simulink model "ContoleLateralApplication_atual"  (R2021a)
settings: Solver=ode23tb  StartTime=0.0  StopTime=TME.Simulation  FixedStep=.001  RelTol=1e-3  EnableMultiTasking=on
StartFcn:
  | %tic
StopFcn:
  | %toc
model workspace (MAT data in the model file):
  A_mu = 10
  B_reff = 8.386
  Cz = 7766.25
  DCT_Param.Transmission.Ratios = [3.78 2.18 1.43 1.03 0.935 0.84]
  DCT_Param.Transmission.Shaft_Inertia_Odd = 0.0023
  DCT_Param.Transmission.Shaft_Inertia_Even = 0.0009
  DCT_Param.Transmission.Shaft_Inertia_Output = 0.008
  DCT_Param.Transmission.Gear_Inertia = 0.001
  DCT_Param.Transmission.Gear_Efficiency = 0.94
  DCT_Param.Transmission.Gear_Ang_Vel_Thr = 0.01
  DCT_Param.Transmission.Shaft_Velocity_Odd = 0
  DCT_Param.Transmission.Shaft_Velocity_Even = 0
  DCT_Param.Transmission.Shaft_Velocity_Output = 0
  DCT_Param.Transmission.Gear_Initial_Velocity = 0
  DCT_Param.Transmission.Abstract.Compliance = 100000
  DCT_Param.Transmission.Abstract.Damping = 10000
  DCT_Param.Transmission.Abstract.Ratio_Time_Const = 0.05
  DCT_Param.Transmission.Abstract.Shift_Gear_Delay = 25
  DCT_Param.Clutch.Torque_Radius = 130
  DCT_Param.Clutch.Num_Friction_Surfaces = 4
  DCT_Param.Clutch.Engagement_Piston_Area = 0.001
  DCT_Param.Clutch.Kinetic_Friction_Coeff = 0.3
  DCT_Param.Clutch.Static_Friction_Coeff = 0.31
  DCT_Param.Clutch.Derating_Factor = 1
  DCT_Param.Clutch.Clutch_Velocity_Tolerance = 0.001
  DCT_Param.Clutch.Threshold_Pressure = 1
  DCT_Param.Clutch.Drag_Torque_Coeff = 0
  DCT_Param.Dog_Clutch.Max_Torque = 1000
  DCT_Param.Dog_Clutch.Teeth_Mean_Radius = 50
  DCT_Param.Dog_Clutch.Tooth_Height = 10
  DCT_Param.Dog_Clutch.Ring_Hub_Clearance = 3
  DCT_Param.Dog_Clutch.Ring_Stop_Stiffness = 1000000
  DCT_Param.Dog_Clutch.Ring_Stop_Damping = 1000
  DCT_Param.Dog_Clutch.Shift_Linkage_Damping = 100
  DCT_Param.Dog_Clutch.Max_Engage_Velocity = 1000000
  DCT_Param.Dog_Clutch.Tooth_Engage_Overlap = 3
  DCT_Param.Vehicle.Mass = 1600
  DCT_Param.Vehicle.Wheels_Per_Axle = 2
  DCT_Param.Vehicle.Distance_CG_FrontAxle = 1.7
  DCT_Param.Vehicle.Distance_CG_RearAxle = 2
  DCT_Param.Vehicle.Distance_CG_Ground = 0.5
  DCT_Param.Vehicle.Frontal_Area = 3
  DCT_Param.Vehicle.Aero_Drag_Coeff = 0.4
  DCT_Param.Vehicle.Initial_Velocity = 0
  DCT_Param.Vehicle.Final_Drive_Ratio = 3.7
  DCT_Param.Vehicle.Final_Drive_Efficiency = 0.86
  DCT_Param.Vehicle.Final_Drive_Vel_Thresh = 0.01
  DCT_Param.Vehicle.Side_Shaft_Inertia = 0.01
  DCT_Param.Vehicle.Side_Shaft_Initial_Velocity = 0
  DCT_Param.Vehicle.Tire.Radius = 0.312
  DCT_Param.Vehicle.Tire.Inertia = 0.5
  DCT_Param.Vehicle.Tire.Initial_Velocity = 0
  DCT_Param.Vehicle.Tire.Slip_Vel_Thresh = 0.1
  DCT_Param.Vehicle.Tire.Nominal_Vertical_Load = 4000
  DCT_Param.Vehicle.Tire.C_Coeff = 1.685
  DCT_Param.Vehicle.Tire.D_Coeff = [1.21 -0.037]
  DCT_Param.Vehicle.Tire.E_Coeff = [0.344 0.095 -0.02 0]
  DCT_Param.Vehicle.Tire.BCD_Coeff = [21.51 -0.163 0.245]
  DCT_Param.Vehicle.Tire.H_Coeff = [-0.002 0.002]
  DCT_Param.Vehicle.Tire.V_Coeff = [0 0]
  DCT_Param.ICE.Max_Power = 100000
  DCT_Param.ICE.Speed_At_Max_Power = 5500
  DCT_Param.ICE.Max_Speed = 7000
  DCT_Param.ICE.Stall_Speed = 200
  DCT_Param.ICE.Shaft_Inertia = 0.2
  DCT_Param.ICE.Initial_Velocity = 800
  DCT_Param.ICE.Idle_Ref_Spd = 800
  DCT_Param.ICE.Engine_Time_Constant = 0.2
  DCT_Param.ICE.Initial_Normalized_Throttle = 0
  DCT_Param.ICE.Speed_Threshold = 20
  DCT_Param.ICE.FC.Speed_Vector = [0 368.421052632 736.842105263 1105.26315789 1473.68421053 1842.10526316 2210.52631579 2578.94736842 2947.36842105 3315.78947368 3684.21052632 4052.63157895 4421.05263158 4789.47368421 5157.89473684 5526.31578947 5894.73684211 6263.15789474 6631.57894737 7000]
  DCT_Param.ICE.FC.Torque_Vector = [0 10.5263157895 21.0526315789 31.5789473684 42.1052631579 52.6315789474 63.1578947368 73.6842105263 84.2105263158 94.7368421053 105.263157895 115.789473684 126.315789474 136.842105263 147.368421053 157.894736842 168.421052632 178.947368421 189.473684211 200]
  DCT_Param.ICE.FC.Consumption_Table = [0.262945178015 0.225304787522 0.201465019624 0.191425874321 0.195187351614 0.212749451502 0.244112173984 0.289275519063 0.348239486736 0.421004077004 0.507569289868 0.607935125326 ... (400 elements, 20x20)]
  DCT_Param.Shift_Map_Example.Pedal_Positions = [0.1 0.4 0.5 0.9]
  DCT_Param.Shift_Map_Example.Upshift_Speeds = [11  20  26  34.5  43; 14  26  35  44.5  55; 17  31  42  52.5  65; 21  39  52  66.5  80]
  DCT_Param.Shift_Map_Example.Downshift_Speeds = [8.9  17  23.6  32.4  40.8; 11.5  22.7  32  41.6  52.2; 14  27  38.1  50  62; 18  33  48  62.6  76.2]
  DCT_Param.Shift_Map_ORIG.Pedal_Positions = [0.1 0.4 0.5 0.9]
  DCT_Param.Shift_Map_ORIG.Upshift_Speeds = [11.5  23.5  35.5  45.5  55.5; 14.5  26.5  38.5  48.5  58.5; 17.5  29.5  41.5  51.5  61.5; 20.5  32.5  44.5  54.5  64.5]
  DCT_Param.Shift_Map_ORIG.Downshift_Speeds = [8.5  20.5  32.5  42.5  52.5; 11.5  23.5  35.5  45.5  55.5; 14.5  26.5  38.5  48.5  58.5; 17.5  29.5  41.5  51.5  61.5]
  DCT_Param.Shift_Map_OPT.Pedal_Positions = [0.1 0.4 0.5 0.9]
  DCT_Param.Shift_Map_OPT.Upshift_Speeds = [17.8469  29.8469  35.8159  41.2981  46.3004; 19.2469  33.9778  43.9778  53.9778  63.9778; 24.5469  41.9778  62.1778  78.5778  106.9778; 27.5469  59.3778  99.0445  109.0445  119.0445]
  DCT_Param.Shift_Map_OPT.Downshift_Speeds = [14.8469  26.8469  32.8159  38.2981  43.3004; 16.2469  30.9778  40.9778  50.9778  60.9778; 21.5469  38.9778  59.1778  75.5778  103.9778; 24.5469  56.3778  96.0445  106.0445  116.0445]
  DCT_Param.Shift_Map.Pedal_Positions = [0.1 0.4 0.5 0.9]
  DCT_Param.Shift_Map.Upshift_Speeds = [11.5  23.5  35.5  45.5  55.5; 14.5  26.5  38.5  48.5  58.5; 17.5  29.5  41.5  51.5  61.5; 20.5  32.5  44.5  54.5  64.5]
  DCT_Param.Shift_Map.Downshift_Speeds = [8.5  20.5  32.5  42.5  52.5; 11.5  23.5  35.5  45.5  55.5; 14.5  26.5  38.5  48.5  58.5; 17.5  29.5  41.5  51.5  61.5]
  DCT_Param.Control.Clutch.Min_Lock_Pressure = 2000000
  DCT_Param.Control.Clutch.Max_Lock_Pressure = 5000000
  DCT_Param.Control.Clutch.Max_Unlock_Pressure = 500000
  DCT_Param.Control.Engine_Start_RPM = 800
  DCT_Param.Control.Engine_Stop_RPM = 790
  DCT_Param.Control.Mode_Logic_TS = 0.1
  DCT_Param.Control.ICE.Kp = 0.02
  DCT_Param.Control.ICE.Ki = 0.01
  DCT_Param.Control.Gen.Kp = 10
  DCT_Param.Control.Gen.Ki = 3
  DCT_Param.Control.Mot.Kp = 500
  DCT_Param.Control.Mot.Ki = 300
  DCT_Param.Control.Veh_Spd.Kp = 0.02
  DCT_Param.Control.Veh_Spd.Ki = 0.04
  DCT_Param.Driver.Kp = 400
  DCT_Param.Driver.Ki = 0.001
  DCT_Param.Driver.Pedal_Filter_Const = 0.01
  DCT_Param.Dog_Clutches.Pulse_Delay = 50
  DCT_Param.Dog_Clutches.Pulse_Length = 20
  DCT_Param.Animation.Teeth_Ratios = [0.338461538462 0.555555555556 0.916666666667 0.96 1.17948717949 1.92307692308]
  DCT_Param.Animation.Teeth_Ratios_Reverse = [0.458333333333 0.75]
  DCT_Param.Shift_Map_OPT506.Pedal_Positions = [0.1 0.4 0.5 0.9]
  DCT_Param.Shift_Map_OPT506.Upshift_Speeds = [18  30.2  48.3  67.3322  77.3429; 20.1  36.85  66.6178  76.7537  86.7537; 21.1  40.25  71.0189  81.0189  91.7873; 24.1  63.75  80.7523  105.9489  115.9489]
  DCT_Param.Shift_Map_OPT506.Downshift_Speeds = [15  27.2  45.3  64.3322  74.3429; 17.1  33.85  63.6178  73.7537  83.7537; 18.1  37.25  68.0189  78.0189  88.7873; 21.1  60.75  77.7523  102.9489  112.9489]
  DCT_Param.Shift_Map_OPTAbsRea176.Pedal_Positions = [0.1 0.4 0.5 0.9]
  DCT_Param.Shift_Map_OPTAbsRea176.Upshift_Speeds = [17.8469  29.8469  35.7875  44.0901  49.4243; 18.9219  34.1312  45.8256  59.7585  69.7585; 32.1719  43.4585  53.51  103.2151  114.6401; 35.1719  59.2585  99.5217  109.5217  119.5217]
  DCT_Param.Shift_Map_OPTAbsRea176.Downshift_Speeds = [14.8469  26.8469  32.7875  41.0901  46.4243; 15.9219  31.1312  42.8256  56.7585  66.7585; 29.1719  40.4585  50.51  100.2151  111.6401; 32.1719  56.2585  96.5217  106.5217  116.5217]
  DLCXref = [0 6 7 14 33.5 34 42 50 60]
  DLCYref = [0 0 -4.5 -4 -3.75 1.5 0.5 0 0]
  D_reff = 0.25826
  Downshift_Speeds = [9.5625  23.0625  36.5625  47.8125  59.0625  68.90625  78.75; 12.9375  26.4375  39.9375  51.1875  62.4375  72.84375  83.25; 16.3125  29.8125  43.3125  54.5625  65.8125  76.78125  87.75; 19.6875  33.1875  46.6875  57.9375  69.1875  80.71875  92.25]
  EngRevLim = 7000
  Pedal_Positions = [0.1 0.4 0.5 0.9]
  SUS.Stiffness = 24000
  SUS.Damping.Constant = 1262
  SUS.Damping.Rebound = [4040 4950 2883 2043]
  SUS.Damping.Compression = [3600 3420 1863 1472]
  SUS.PistonSpeed = [0.05 0.1 0.3 0.6]
  SUS.UnsprungMass.Fr = 21.0693333333
  SUS.UnsprungMass.Rr = 21.0693333333
  Upshift_Speeds = [12.9375  26.4375  39.9375  51.1875  62.4375  72.84375  83.25; 16.3125  29.8125  43.3125  54.5625  65.8125  76.78125  87.75; 19.6875  33.1875  46.6875  57.9375  69.1875  80.71875  92.25; 33  52.5  77.25  100.5  138.75  161.875  185]
  VEH.Mass = 1181
  VEH.StaticNormalFrontLoad.FR = 264.666666667
  VEH.StaticNormalFrontLoad.FL = 264.666666667
  VEH.StaticNormalRearLoad.RR = 322
  VEH.StaticNormalRearLoad.RL = 322
  VEH.WheelBase = 3.075
  VEH.FrontAxlePositionfromCG = 1.515
  VEH.RearAxlePositionfromCG = 1.504
  VEH.HeightCG = 0.134
  VEH.FrontalArea = 2.11
  VEH.DragCoefficient = 0.33
  VEH.NumberOfWheelsPerAxle = 2
  VEH.Thread.FR = 1.705
  VEH.Thread.RR = 1.705
  VEH.PitchMomentInertia = 1922.66666667
  VEH.RollMomentInertia = 432.333333333
  VEH.YawMomentInertia = 2066
  VEH.SteeringRatio = 18
  VEH.TrackWidth = 1.922
  VEH.SprungMass = 1096.72266667
  VEH.InitialLongPosition = 0
  VEH.InitialLatPosition = 0
  VEH.InitialVertPosition = 0
  VEH.InitialRollAngle = 0
  VEH.InitialPitchAngle = 0
  VEH.InitialYawAngle = 0
  VEH.InitialLongVel = 0
  VEH.InitialLatVel = 0
  VEH.InitialVertVel = 0
  VEH.InitialRollRate = 0
  VEH.InitialPitchRate = 0
  VEH.InitialYawRate = 0
  V_o = 16.7
  V_xlow = 1
  WH.Tire.Radius.Front = 0.384
  WH.Tire.Radius.Rear = 0.401
  WH.Tire.Sidewall = 0.245
  WH.Tire.RollingResistCoeff = 0.0103
  WH.Tire.Magic.B = 10
  WH.Tire.Magic.C = 1.9
  WH.Tire.Magic.D = 1
  WH.Tire.Magic.E = 0.97
  WH.Tire.Magic.Bx = 12
  WH.Tire.Magic.Cx = 1.9
  WH.Tire.Magic.Dx = 0.72
  WH.Tire.Magic.Ex = 0.95
  WH.Tire.Magic.By = 12
  WH.Tire.Magic.Cy = 1.3
  WH.Tire.Magic.Dy = 0.75
  WH.Tire.Magic.Ey = 0.2
  WH.Tire.Front.Ky = 40000
  WH.Tire.Rear.Ky = 40000
  WH.Tire.Kz = 320000
  WH.Tire.Damping = 100
  WH.Inertia = 1.00333333333
  WH.Mass = 11.4333333333
  WH.DampingCoefficient = 0.01
  WH.VelocityTol = 0.1
  a = 1.4
  alpha_max = 1.5
  alpha_min = -1.5
  b = 1.8
  c_zo = 209651
  epsilon = 0.1
  h = 0.134
  path.ISO3888p2.x = [0 2 12 25.5 36.5 49 61]
  path.ISO3888p2.y = [0 0 0 3.725 3.725 0 0]
  path.ISO3888p2.ylb = [1.225 1.225 1.225 4.725 4.725 1.5 1.5]
  path.ISO3888p2.yrb = [-1.225 -1.225 -1.225 2.225 2.225 -1.5 -1.5]
  path.CUSC.x = [10.668 21.336 36.576 54.864 73.152]
  path.CUSC.y = [0 0 5.1816 0 0]
  path.CUSC.ylb = [1.2192 1.2192 7.0104 1.8288 1.8288]
  path.CUSC.yrb = [-1.2192 -1.2192 3.3528 -1.8288 -1.8288]
  pio = 220000
  q_Fcx = 0
  q_Fz2 = 15.4
  q_Fzy = 0
  q_reo = 0.9974
  q_sx1 = -0.007764
  q_sx10 = 0.2824
  q_sx11 = 5.349
  q_sx12 = 0
  q_sx13 = 0
  q_sx14 = 0
  q_sx2 = 1.1915
  q_sx3 = 0.013948
  q_sx4 = 4.912
  q_sx5 = 1.02
  q_sx6 = 22.83
  q_sx7 = 0.7104
  q_sx8 = -0.023393
  q_sx9 = 0.6581
  q_sy1 = 0.00702
  q_sy2 = 0
  q_sy3 = 0.001515
  q_sy4 = 8.514e-05
  q_sy5 = 0
  q_sy6 = 0
  q_sy7 = 0.9008
  q_sy8 = -0.4089
  q_v1 = 0.0007742
  q_v2 = 0.04667
  r_Bx1 = 12.531
  r_Bx2 = 9.532
  r_Bx3 = 0
  r_By1 = 10.615
  r_By2 = 7.705
  r_By3 = 3.433e-06
  r_By4 = 0
  r_Cx1 = 1.019
  r_Cy1 = 1.0585
  r_Ex1 = -0.4487
  r_Ex2 = -0.4726
  r_Ey1 = 0.3132
  r_Ey2 = 7.63e-06
  r_Hx1 = 0.0002374
  r_Hy1 = 0.011646
  r_Hy2 = 7.63e-06
  r_Vy1 = 0.05654
  r_Vy2 = 7.63e-06
  r_Vy3 = 0
  r_Vy4 = 99.9
  r_Vy5 = 2
  r_Vy6 = 15.814
  r_o = 0.3135
  vehWidth = 2
  w = 1
values from neighbouring files (symbols this model uses):
  C1 = 1.2801    [Data_ControleLateral_atual.m]
  C2 = 23.99    [Data_ControleLateral_atual.m]
  C3 = 0.52    [Data_ControleLateral_atual.m]
undefined symbols (not defined in the file or in its folder): Disabled, EV, GND, MTR, Right, SENSOR, STEER, WHL
libraries: autolibutils x5, vehdynlibscenariocommon x5, autolibshared x5, sim3dlib x4, vehdynlibtirecommon x2, autolibmappedmotor x2, vehdynlibviscommon x2, vehdynlibsteering x1, pid_lib x1, vehdynlibdriver x1, vehdynlibsens x1, sharedtransform x1
(part 1 of 6)
settings Model: SimulationMode=accelerator  NumberOfSteps=10  OrderedModelArguments=off  Creator=The MathWorks, Inc.  LastModifiedBy=Luiza
settings SolverCC: ZeroCrossAlgorithm=Adaptive  AlgebraicLoopSolver=TrustRegion  AutoInsertRateTranBlk=on  InsertRTBMode=Never (minimum delay)  DecoupledContinuousIntegration=on  MinimalZcImpactIntegration=on
settings OptimizationCC: EfficientMapNaN2IntZero=off
settings DebuggingCC: SignalInfNanChecking=error  ArtificialAlgebraicLoopMsg=none  MaskedZcDiagnostic=none  IgnoredZcDiagnostic=none  ModelReferenceExtraNoncontSigs=none  PregeneratedLibrarySubsystemCodeDiagnostic=none  SFMachineParentedDataDiag=warning  ArithmeticOperatorsInVariantConditions=warning
settings HardwareCC: TargetBitPerPointer=64  TargetBitPerSizeT=64  TargetBitPerPtrDiffT=64  TargetLongLongMode=on  TargetIntDivRoundTo=Zero  TargetEndianess=LittleEndian  TargetWordSize=64  TargetHWDeviceType=MATLAB Host  ProdEqTarget=off
settings ModelReferenceCC: UpdateModelReferenceTargets=IfOutOfDate  EnableParallelModelReferenceBuilds=on  ModelReferenceMinAlgLoopOccurrences=on  PropagateSignalLabelsOutOfModel=off
settings SFSimCC: SimUseLocalCustomCode=off  CustomCodeUndefinedFunction=UseInterfaceOnly
settings CodeAppCC: MaxIdLength=128
settings GRTTargetCC: TargetLangStandard=C89/C90 (ANSI)  CombineOutputUpdateFcns=off  GRTInterface=on

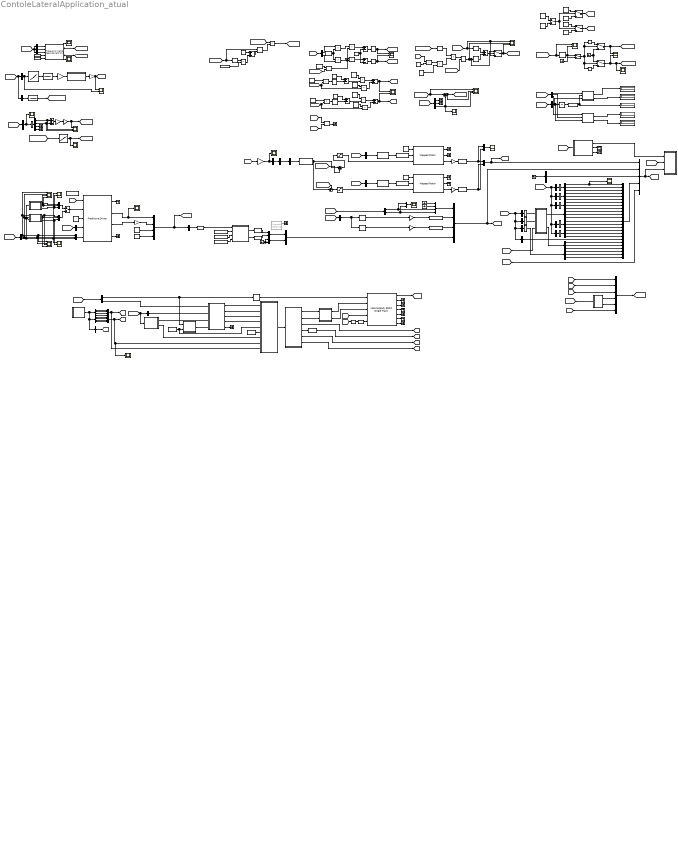
== system ContoleLateralApplication_atual ==
  note: Pista
  note: Avaliação
  note: Skid Pad / Slalom
  note: Steering System
  note: Driveline
  note: Powertrain
  note: Copyright 2018 The MathWorks, Inc.
  note: Copyright 2017-2018 The MathWorks, Inc.
  note: Taxa de guinada máxima
  note: Diferença entre guinadas
  note: GUINADA DESEJADA
      |
      | Variaveis necessárias:
      | Velocidade CG (vCG) - gps; velo. média rodas dianteiras (OK)
      | Lr + Lf - distancia entre os eixos traseiro e frontal (OK)
      | Ku - taxa de guinada desejada (OK)
      | Cy,f / Cy,r - rigidez dos pneus dianteiros e traseiros na curva (OK)
      | m - massa (OK)
      | Delta minusculo - angulo direçao (OK)
      |
      | GUINADA MÁXIMA
      |
      | Sigma: fator de ajustabilidade; necessita de teste para definido, varia cm o pavimento
      | Micro g: coeficiente de atrito (padrao);
      | vCG : velo, centro de gravidade
  note: Taxa de guinada desejada
  note: Variáveis
  note: ControladorVT
  note: APPS
  note: IMU
  note: Volante
  note: Sensores
  note: Coeficiente de atrito
  note: SLIP RATIO
      |
      | COEFICIENTE DE ATRITO
  Abs{,1..5} (6 alike) : Abs
  Acc to Torque Request : Gain  Gain=MTR.MaxTorque*0.01
  AccelCmd% : Gain  Gain=100
  Accelerometer : Scope
  Add : Sum
  Add1 : Sum
  Add{2..8} (7 alike) : Sum  Inputs=+-
  AngVolante-> AngRoda : Lookup_n-D  NumberOfTableDimensions=1  BreakpointsForDimension1=STEER.Volante  Table=SENSOR.SteerAvg  InternalRulePriority=Speed  RndMeth=Simplest  InputSameDT=on
  Axle Forces : Subsystem  Variant=on  VariantControlMode=label  LabelModeActiveChoice=1
  Bus Creator : BusCreator  Inputs=25
  Bus Creator1 : BusCreator  Inputs=4
  Bus Creator10 : BusCreator  Inputs=1
  Bus Creator11 : BusCreator  Inputs=4
  Bus Creator13 : BusCreator  Inputs=2
  Bus Creator2 : BusCreator  Inputs=5
  Bus Creator3 : BusCreator  Inputs=6
  Bus Creator4 : BusCreator  Inputs=1
  Bus Creator5 : BusCreator  Inputs=2
  Bus Creator9 : BusCreator  Inputs=1
  Bus Selector : BusSelector  OutputSignals=ECU.EngTrqCmd
  Bus Selector1 : BusSelector  OutputSignals=InertFrm.Cg.Disp.X,InertFrm.Cg.Disp.Y,InertFrm.Cg.Disp.Z  OutputAsBus=on
  Bus Selector10 : BusSelector  OutputSignals=Gnd.z.G_FL_z,Gnd.z.G_FR_z,Gnd.z.G_RL_z,Gnd.z.G_RR_z
  Bus Selector11 : BusSelector  OutputSignals=Wind
  Bus Selector12 : BusSelector  OutputSignals=Gnd.mu.mu_FL,Gnd.mu.mu_FR,Gnd.mu.mu_RL,Gnd.mu.mu_RR
  Bus Selector13 : BusSelector  OutputSignals=WhlAng,AxlTrq
  Bus Selector14 : BusSelector  OutputSignals=Steer
  Bus Selector15 : BusSelector  OutputSignals=omega
  Bus Selector16 : BusSelector  OutputSignals=BdyFrm.Cg.AngVel.r
  Bus Selector17 : BusSelector  OutputSignals=LeftMtrTrq,RghtMtrTrq
  Bus Selector18 : BusSelector  OutputSignals=LeftMtrSpd
  Bus Selector19 : BusSelector  OutputSignals=RghtMtrSpd
  Bus Selector2 : BusSelector  OutputSignals=InertFrm.Cg.Vel.Xdot,InertFrm.Cg.Vel.Ydot,InertFrm.Cg.Vel.Zdot  OutputAsBus=on
  Bus Selector20 : BusSelector  OutputSignals=Chassis.psi,Chassis.Y,Chassis.X
  Bus Selector21 : BusSelector  OutputSignals=LeftMtrSpd,RghtMtrSpd
  Bus Selector23 : BusSelector  OutputSignals=Steer
  Bus Selector25 : BusSelector  OutputSignals=Accel
  Bus Selector26 : BusSelector  OutputSignals=BdyFrm.Cg.Vel.xdot
  Bus Selector27 : BusSelector  OutputSignals=BdyFrm.Cg.AngVel  OutputAsBus=on
  Bus Selector28 : BusSelector  OutputSignals=BdyFrm.Cg.Acc.ax,BdyFrm.Cg.Acc.ay,BdyFrm.Cg.Acc.az  OutputAsBus=on
  Bus Selector29 : BusSelector  OutputSignals=BdyFrm.Cg.Acc.xddot,BdyFrm.Cg.Acc.yddot,BdyFrm.Cg.Acc.zddot  OutputAsBus=on
  Bus Selector3 : BusSelector  OutputSignals=BdyFrm.Cg.Acc.ax,BdyFrm.Cg.Acc.ay,BdyFrm.Cg.Acc.az  OutputAsBus=on
  Bus Selector31 : BusSelector  OutputSignals=Chassis.X,Chassis.Y,Chassis.psi
  Bus Selector32 : BusSelector  OutputSignals=omega
  Bus Selector33 : BusSelector  OutputSignals=BdyFrm.Cg.Vel.xdot  OutputAsBus=on
  Bus Selector4 : BusSelector  OutputSignals=InertFrm.Cg.Ang.phi,InertFrm.Cg.Ang.theta,InertFrm.Cg.Ang.psi  OutputAsBus=on
  Bus Selector5 : BusSelector  OutputSignals=BdyFrm.Cg.AngVel.p,BdyFrm.Cg.AngVel.q,BdyFrm.Cg.AngVel.r  OutputAsBus=on
  Bus Selector6 : BusSelector  OutputSignals=InertFrm.Geom.Disp.X,InertFrm.Geom.Disp.Y,InertFrm.Geom.Disp.Z  OutputAsBus=on
  Bus Selector7 : BusSelector  OutputSignals=InertFrm.Geom.Vel.Xdot,InertFrm.Geom.Vel.Ydot,InertFrm.Geom.Vel.Zdot  OutputAsBus=on
  Bus Selector8 : BusSelector  OutputSignals=BdyFrm.Geom.Ang.Beta
  Bus Selector9 : BusSelector  OutputSignals=BdyFrm.Cg.Vel.xdot,BdyFrm.Cg.Vel.ydot,BdyFrm.Cg.Vel.zdot  OutputAsBus=on
  Bus to Vector{,1..8} (9 alike) : BusToVector
  Constant : Constant  Value=76
  Constant1 : vehdynlibtirecommon/Constant  const=180000  numWheels=4
      settings: SourceProductBaseCode=VE
  Constant10 : Constant  Value=C3
  Constant11 : Constant  Value=STEER.Volante
  Constant12 : Constant  Value=STEER.Left
  Constant13 : Constant  Value=[0 0 0]
  Constant14 : Constant  Value=0
  Constant15 : Constant  Value=100
  Constant16 : Constant  Value=[0 0 9.78]
  Constant17 : Constant
  Constant18 : Constant  Value=C3
  Constant19 : Constant
  Constant2 : Constant  Value=76
  Constant20 : Constant  Value=C1
  Constant21 : Constant  Value=EV.InitialLongVel
  Constant22 : Constant  Value=0
  Constant23 : Constant  Value=-C2
  Constant24 : Constant  Value=9.1
  Constant25 : Constant  Value=1.3
  Constant26 : Constant  Value=1.1
  Constant27 : Constant  Value=8.7
  Constant3 : vehdynlibtirecommon/Constant  const=0  numWheels=4
      settings: SourceProductBaseCode=VE
  Constant4 : Constant  Value=2*pi/60
  Constant5 : Constant  Value=0.2566
  Constant6 : Constant
  Constant7 : Constant  Value=C1
  Constant8 : Constant  Value=-C2
  Constant9 : Constant  Value=STEER.Right
  Cálculo do Skidpad : MATLAB Function  TreatAsAtomicUnit=on
  Cálculo do Slalom : MATLAB Function  TreatAsAtomicUnit=on
  Demux{,1..7,9} (9 alike) : Demux  Outputs=3
  Demux8 : Demux
  Distância Percorrida : Display
  Divide : Product  Inputs=*/
  Divide1 : Product  Inputs=*/
  Divide2 : Product  Inputs=*/
  Diâmetro : Display
  Electronic Throttle Actuator Dynamics : autolibutils/Cont LPF  wc=2*pi/.0085  aMode=2
      settings: SourceProductBaseCode=PW,DR,MT,UV,VE
  Engine Response : autolibutils/Cont LPF  wc=40*2*pi  aMode=2
      settings: SourceProductBaseCode=PW,DR,MT,UV,VE
  Engine Response1 : autolibutils/Cont LPF  wc=40*2*pi  aMode=2
      settings: SourceProductBaseCode=PW,DR,MT,UV,VE
  Entre-Eixos : Constant  Value=EV.WheelBase
  Environment : Subsystem
      mask Display: disp('Environment')
  Fator de ajustabilidade : Constant
  For 3D Visualization : MATLAB Function  TreatAsAtomicUnit=on  mask{trackW=VEH.TrackWidth, wheelB=VEH.FrontAxlePositionfromCG+VEH.RearAxlePositionfromCG}
      mask prompts: trackW "Vehicle track width, trackW [m]:"; wheelB "Vehicle wheelbase, wheelB [m]:"
      mask help: This block converts wheel ground height information into estimates of vehicle pitch, roll angles and vertical height in order to help in the visualization 3DOF based simulations with changes in terrain. Note that the resulting signals are only used as a visualization aid and do not account for the physical affects of the vehicle interacting with variable terrain or changes in orientation.
  Gain : Gain  Gain=9
  Gain1 : Gain  Gain=9*.9
  Gain2 : Gain  Gain=9*.9
  Gain3 : Gain  Gain=9
  Gain5 : Gain  Gain=0.1
  Gain6 : Gain  Gain=819.2
  Gain9 : Gain  Gain=0.5
  Gravidade : Constant  Value=9.81
  Ground{,1..4,6} (6 alike) : Ground
  Gyroscope : Scope
  Integrator1 : Integrator
  Kinematic Steering : vehdynlibsteering/Kinematic Steering  Commented=on  StrgType=Ackerman  StrgRatioType=Constant  Loc=Front  NrmlFctr=1  TrckWdth=EV.TrackWidth(1)  WhlBase=EV.WheelBase  Db=0  StrgRng=1.963  StrgAngBpts="[-2.1 -1.68 -1.26 -0.87 -0.41  0 0.41 0.87 1.26 1.68 2.1]"  StrgRatioTbl=|  StrgRatio=3.6  StrgArmLngth=0.082  RckCsLngth=0.4065  TieRodLngth=0.35562  D=0.080  PnnRadius=0.035336  PnnRadiusTbl="[0.0055    0.0055    0.0056    0.0057    0.0057    0.0057    0.0057    0.0057    0.0056    0.0055    0.0055]*6.5"  RodLngth=0.1  ParaArmLngth=0.9  aMode=2
      | [3.75   3.75  3.750   13.1250   13.0000   13.0000   13.0000   13.1250   13.2500   13.3750   13.5000
      | ]
  Kinematic Steering V2 : MATLAB Function  TreatAsAtomicUnit=on
  Ku : Constant  Value=(EV.RearAxlePositionfromCG*EV.Mass)/(EV.CornerStiffFront *EV.WheelBase)-(EV.FrontAxlePositionfromCG*EV.Mass)/(EV.CornerStiffRear*EV.WheelBase)
  Manual Switch : ManualSwitch
  Manual Switch1 : ManualSwitch
  Manual Switch3 : ManualSwitch
  "Mapped Left Motor " : autolibmappedmotor/Mapped Motor  port_config=Speed  param_by=Tabulated torque-speed envelope  w_t=MTR.Speed  T_t=MTR.Torque*MTR.Overpower  torque_max=.1  power_max=30  Tc=0.05  param_loss=Single efficiency measurement  eff=100  w_eff=375  T_eff=0.08  Piron=0  Pbase=0  w_eff_bp=[-8000 -4000 0 4000 8000]  T_eff_bp=[0 0.03 0.06 0.09]  Temp_eff_bp=[233.15 293.15 373.15]  losses_table=[1.49 1.67 2.21 3.10; 0.42 0.69 1.14 2.03; 0.06 0.24 0.78 1.68; 0.42 0.69 1.14 2.03; 1.49 1.67 2.21 3.10]  losses_table_3d=cat(3,1.05*[1.49 1.67 2.21 3.10; 0.42 0.69 1.14 2.03; 0.06 0.24 0.78 1.68; 0.42 0.69 1.14 2.03; 1.49 1.67 2.21 3.10],[1.49 1.67 2.21 3.10; 0.42 0.69 1.14 2.03; 0.06 0.24 0.78 1.68; 0.42 0.69 1.14 2.03; 1.49 1.67 2.21 3.10],1.03*[1.49 1.67 2.21 3.10; 0.42 0.69 1.14 2.03; 0.06 0.24 0.78 1.68; 0.42 0.69 1.14 2.03; 1.49 1.67 2.21 3.10])  efficiency_table=[95 95 95 95; 95 95 95 95; 95 95 95 95; 95 95 95 95; 95 95 95 95]  efficiency_table_3d=cat(3,90*ones(5,4),95*ones(5,4),92*ones(5,4))  J=5e-6  b=1e-5  omega_o=0  T_t_extended=[0.35 22.4 23.8 26.95 31.5 37.1 45.85 45.85 45.85 37.1 31.5 26.95 23.8 22.4 0.35]  w_t_extended=[-943 -942 -880 -775 -670 -565 -461 0 461 565 670 775 880 942 943]  KLossIron=0  KLossCopper=0  x_w_eff_vec=[-8000 -4000 0 4000 8000]  x_T_eff_vec=[-0.09 -0.06 -0.03 0 0.03 0.06 0.09]  x_tmp_eff_vec=[233.15 293.15 373.15]  x_losses_mat=[3.1 2.21 1.67 1.49 1.67 2.21 3.1;2.03 1.14 0.69 0.42 0.69 1.14 2.03;1.68 0.78 0.24 0.06 0.24 0.78 1.68;2.03 1.14 0.69 0.42 0.69 1.14 2.03;3.1 2.21 1.67 1.49 1.67 2.21 3.1]  x_losses_mat_3d=cat(3,[3.255 2.3205 1.7535 1.5645 1.7535 2.3205 3.255;2.1315 1.197 0.7245 0.441 0.7245 1.197 2.1315;1.764 0.819 0.252 0.063 0.252 0.819 1.764;2.1315 1.197 0.7245 0.441 0.7245 1.197 2.1315;3.255 2.3205 1.7535 1.5645 1.7535 2.3205 3.255],[3.1 2.21 1.67 1.49 1.67 2.21 3.1;2.03 1.14 0.69 0.42 0.69 1.14 2.03;1.68 0.78 0.24 0.06 0.24 0.78 1.68;2.03 1.14 0.69 0.42 0.69 1.14 2.03;3.1 2.21 1.67 1.49 1.67 2.21 3.1],[3.193 2.2763 1.7201 1.5347 1.7201 2.2763 3.193;2.0909 1.1742 0.7107 0.4326 0.7107 1.1742 2.0909;1.7304 0.8034 0.2472 0.0618 0.2472 0.8034 1.7304;2.0909 1.1742 0.7107 0.4326 0.7107 1.1742 2.0909;3.193 2.2763 1.7201 1.5347 1.7201 2.2763 3.193])  CalLossMapData={}  CalLossWithTempMapData={}  aMode=2  RefBlkName='autolibmappedmotor/Mapped Motor'
      settings: SourceProductBaseCode=PW,DR,MT,UV,VE
  "Mapped Right Motor " : autolibmappedmotor/Mapped Motor  port_config=Speed  param_by=Tabulated torque-speed envelope  w_t=MTR.Speed  T_t=MTR.Torque*MTR.Overpower  torque_max=.1  power_max=30  Tc=0.05  param_loss=Single efficiency measurement  eff=100  w_eff=375  T_eff=0.08  Piron=0  Pbase=0  w_eff_bp=[-8000 -4000 0 4000 8000]  T_eff_bp=[0 0.03 0.06 0.09]  Temp_eff_bp=[233.15 293.15 373.15]  losses_table=[1.49 1.67 2.21 3.10; 0.42 0.69 1.14 2.03; 0.06 0.24 0.78 1.68; 0.42 0.69 1.14 2.03; 1.49 1.67 2.21 3.10]  losses_table_3d=cat(3,1.05*[1.49 1.67 2.21 3.10; 0.42 0.69 1.14 2.03; 0.06 0.24 0.78 1.68; 0.42 0.69 1.14 2.03; 1.49 1.67 2.21 3.10],[1.49 1.67 2.21 3.10; 0.42 0.69 1.14 2.03; 0.06 0.24 0.78 1.68; 0.42 0.69 1.14 2.03; 1.49 1.67 2.21 3.10],1.03*[1.49 1.67 2.21 3.10; 0.42 0.69 1.14 2.03; 0.06 0.24 0.78 1.68; 0.42 0.69 1.14 2.03; 1.49 1.67 2.21 3.10])  efficiency_table=[95 95 95 95; 95 95 95 95; 95 95 95 95; 95 95 95 95; 95 95 95 95]  efficiency_table_3d=cat(3,90*ones(5,4),95*ones(5,4),92*ones(5,4))  J=5e-6  b=1e-5  omega_o=0  T_t_extended=[0.35 22.4 23.8 26.95 31.5 37.1 45.85 45.85 45.85 37.1 31.5 26.95 23.8 22.4 0.35]  w_t_extended=[-943 -942 -880 -775 -670 -565 -461 0 461 565 670 775 880 942 943]  KLossIron=0  KLossCopper=0  x_w_eff_vec=[-8000 -4000 0 4000 8000]  x_T_eff_vec=[-0.09 -0.06 -0.03 0 0.03 0.06 0.09]  x_tmp_eff_vec=[233.15 293.15 373.15]  x_losses_mat=[3.1 2.21 1.67 1.49 1.67 2.21 3.1;2.03 1.14 0.69 0.42 0.69 1.14 2.03;1.68 0.78 0.24 0.06 0.24 0.78 1.68;2.03 1.14 0.69 0.42 0.69 1.14 2.03;3.1 2.21 1.67 1.49 1.67 2.21 3.1]  x_losses_mat_3d=cat(3,[3.255 2.3205 1.7535 1.5645 1.7535 2.3205 3.255;2.1315 1.197 0.7245 0.441 0.7245 1.197 2.1315;1.764 0.819 0.252 0.063 0.252 0.819 1.764;2.1315 1.197 0.7245 0.441 0.7245 1.197 2.1315;3.255 2.3205 1.7535 1.5645 1.7535 2.3205 3.255],[3.1 2.21 1.67 1.49 1.67 2.21 3.1;2.03 1.14 0.69 0.42 0.69 1.14 2.03;1.68 0.78 0.24 0.06 0.24 0.78 1.68;2.03 1.14 0.69 0.42 0.69 1.14 2.03;3.1 2.21 1.67 1.49 1.67 2.21 3.1],[3.193 2.2763 1.7201 1.5347 1.7201 2.2763 3.193;2.0909 1.1742 0.7107 0.4326 0.7107 1.1742 2.0909;1.7304 0.8034 0.2472 0.0618 0.2472 0.8034 1.7304;2.0909 1.1742 0.7107 0.4326 0.7107 1.1742 2.0909;3.193 2.2763 1.7201 1.5347 1.7201 2.2763 3.193])  CalLossMapData={}  CalLossWithTempMapData={}  aMode=2  RefBlkName='autolibmappedmotor/Mapped Motor'
      settings: SourceProductBaseCode=PW,DR,MT,UV,VE
  Math Function : Math  Operator=square  SaturateOnIntegerOverflow=on
  Math Function1 : Math  SaturateOnIntegerOverflow=on
  Math Function2 : Math  SaturateOnIntegerOverflow=on
  Min1 : MinMax  Inputs=2
  PID Controller1 : pid_lib/PID Controller  Controller=PI  Form=Parallel  TimeDomain=Continuous-time  UseExternalTs=off  SampleTime=-1  IntegratorMethod=Forward Euler  FilterMethod=Forward Euler  ControllerParametersSource=internal  P=6.51864262048678  I=43.9160892044863  D=-1.04450033164761  UseFilter=on  N=21.9051072982779  TunerSelectOption=Transfer Function Based (PID Tuner App)  InitialConditionSource=internal  InitialConditionForIntegrator=0  InitialConditionForFilter=0  DifferentiatorICPrevScaledInput=0  ExternalReset=none  TrackingMode=off  Kt=1  LimitOutput=off  SatLimitsSource=internal  UpperSaturationLimit=inf  LowerSaturationLimit=-inf  LinearizeAsGain=on  AntiWindupMode=none  Kb=1  POutMin=[]  POutMax=[]  IOutMin=[]  IOutMax=[]  DOutMin=[]  DOutMax=[]  NOutMin=[]  NOutMax=[]  SumOutMin=[]  SumOutMax=[]  SaturationOutMin=[]  SaturationOutMax=[]  PParamMin=[]  PParamMax=[]  IParamMin=[]  IParamMax=[]  DParamMin=[]  DParamMax=[]  NParamMin=[]  NParamMax=[]  KbParamMin=[]  KbParamMax=[]  KtParamMin=[]  KtParamMax=[]  KbOutMin=[]  KbOutMax=[]  KtOutMin=[]  KtOutMax=[]  IntegratorOutMin=[]  IntegratorOutMax=[]  FilterOutMin=[]  FilterOutMax=[]  SumI1OutMin=[]  SumI1OutMax=[]  SumI2OutMin=[]  SumI2OutMax=[]  SumI3OutMin=[]  SumI3OutMax=[]  SumI4OutMin=[]  SumI4OutMax=[]  SumDOutMin=[]  SumDOutMax=[]  DifferentiatorOutMin=[]  DifferentiatorOutMax=[]  FilterDiffOutCoefMin=[]  FilterDiffOutCoefMax=[]  ReciprocalOutMin=[]  ReciprocalOutMax=[]  SumDenOutMin=[]  SumDenOutMax=[]  SumNumOutMin=[]  SumNumOutMax=[]  DivideOutMin=[]  DivideOutMax=[]  UdiffTsProdOutMin=[]  UdiffTsProdOutMax=[]  NTsProdOutMin=[]  NTsProdOutMax=[]  UintegralTsProdOutMin=[]  UintegralTsProdOutMax=[]  UngainTsProdOutMin=[]  UngainTsProdOutMax=[]  IntegratorContinuousStateAttributes=''  IntegratorStateMustResolveToSignalObject=off  IntegratorRTWStateStorageClass=Auto  FilterContinuousStateAttributes=''  FilterStateMustResolveToSignalObject=off  FilterRTWStateStorageClass=Auto  ParallelPVariant=InternalParameters  IdealPVariant=Disabled  IVariant=InternalParameters  DVariant=Disabled  IntegratorVariant=Continuous  SatVariant=Disabled  AWVariant=Passthrough  PCopyVariant=Disabled  TRVariant=Disabled  FdbkBlocksVariant=Forward  IdealPFdbkVariant=Disabled  SatFdbkVariant=Disabled  DerivativeFilterVariant=Disabled  NVariant=Disabled  NCopyVariant=Disabled_SignalSpec  FilterICVariant=Disabled  IntegratorICVariant=InternalICs  ExternalResetVariant=Disabled  TRSumVariant=Passthrough  SumFdbkVariant=Disabled  SumVariant=Sum_PI  TsampFilterVariant=InternalTs  TsampNgainVariant=Passthrough  TsampIntegralVariant=Passthrough  ExternalSaturationOutDataTypeStr=Inherit: Same as second input
  Pista molhada : Constant  Value=-1
  Pista seca : Constant
  "Posição -> Tensão" : Lookup_n-D  NumberOfTableDimensions=1  BreakpointsForDimension1=SENSOR.APPSAcionado  Table=SENSOR.APPS1  InternalRulePriority=Speed  RndMeth=Simplest  InputSameDT=on
  Predictive Driver1 : vehdynlibdriver/Predictive Driver  extAccelOvr=off  extDecelOvr=off  extAccelHld=off  extDecelHld=off  extAccelZero=off  extDecelZero=off  extSteerOvr=off  extSteerHld=off  extSteerZero=off  cntrlType=PI  cntrlTypeLat=Stanley  shftType=None  coordMode=SAE J670 (Z-down)  velUnits=m/s  angUnits=rad  gearOut=off  steerOut=off  Kp=10  Ki=5  Kff=.1  Kg=0  VehVelVec=[0 100]  KffVec=[.1 .1]  KpVec=[10 10]  KiVec=[5 5]  KgVec=[0 0]  vnom=5  Kaw=1  tauerr=.01  tau=0.1  L=3  Kpt=3000  aR=200  bR=2.5  cR=.5  g=9.81  vecPose=on  dynamMode=off  PositionGainF=2.5  PositionGainR=2.5  YawRateGain=.2  DelayGain=.2  a=0.775  b=0.775  m=2016  Cy_f=25266  Cy_r=70933  I=4013  Ksteer=18  theta=0.523598776  GearInit=0  tShift=.1  pdlVec=[0.1 0.4 0.5 0.9]  upShftTbl=[-1 12.9375 26.4375 39.9375 51.18749999999999 62.4375 72.84375 83.25;-1 16.3125 29.8125 43.3125 54.5624 65.8125 76.78125 87.75;-1 19.6875 33.1875 46.68749999999999 57.9375 69.1875 80.71875 92.25;-1 33 52.5 77.25 100.5 138.75 161.875 185]  dwnShftTbl=[-1 12.9375 26.4375 39.9375 51.18749999999999 62.4375 72.84375 83.25;-1 16.3125 29.8125 43.3125 54.5624 65.8125 76.78125 87.75;-1 19.6875 33.1875 46.68749999999999 57.9375 69.1875 80.71875 92.25;-1 33 52.5 77.25 100.5 138.75 161.875 185]  tClutch=.5  tRev=.5  tPark=120  UpGearVec="[0  1  2  3  4  5  6  7]"  DownGearVec="[1  2  3  4  5  6  7  8]"  aMode=2
      settings: SourceProductBaseCode=VE
  Product{,1..14} (15 alike) : Product
  Raio máximo : Display
  Reference Generator : Subsystem  mask(Reference Generator){manType=Constant Radius, manOverride=off, prevType=Constant Radius, t_start=1, xdot_r=21, xdotUnit=mph, aMode=2, omega_hw=13.5, theta_max=90, t_stop=60, ay_max=.5, ay_stop=on, XGate=174.5, xStart=2, vehW=1.2, lattoff=VEH.InitialLatPosition, latRefbp=DLCXref, latRef=DLCYref, t_sweep=30, theta_hw=90, theta_hw_final=.7, steerF=.7, steerA=90, tdwell=.5, steerDir=off, R=18.25/2, turnDirMask=Right, cr_ay_max=0.5, cr_ay_stop=off, simTime=60, engine3D=Disabled, SceneDesc=Straight road, dt3D=.03, defaultPos=Recommended for scene, X_o=-118, Y_o=3.125, Z_o=0, phi_o=0, theta_o=0, psi_o=0}
      mask prompts: manType "Maneuver"; manOverride "Use maneuver-specific driver, initial position, and scene"; t_start "Maneuver start time, t_start [s]:"; xdot_r "Longitudinal velocity reference, xdot_r:"; xdotUnit "Longitudinal entrance velocity setpoint units, xdotUnit []:"; omega_hw "Handwheel rate, omega_hw [deg/s]:"; theta_max "Maximum handwheel angle, theta_max [deg]:"; t_stop "Steering hold time after max angle reached, t_stop [s]:"; ay_max "Lateral acceleration threshold, ay_max [g]:"; ay_stop "Stop simulation at lateral acceleration threshold"; XGate "Inertial longitudinal position of gate entrance, XGate [m]:"; xStart "Distance after target speed to begin reference, x_start [m]:"; vehW "Vehicle width, vehW [m]:"; lattoff "Lateral offset, latoff [m]:"; latRefbp "Lateral reference position breakpoints [m]:"; latRef "Lateral reference data, latRef [m]:"; t_sweep "Swept time, t_sweep [s]:"; theta_hw "Steering amplitude, theta_hw [deg]"; theta_hw_final "Final frequency, theta_hw_final [Hz]:"; steerF "Steer frequency, steerF [Hz]:"; steerA "Steer amplitude, steerA [deg]:"; tdwell "Dwell time, tdwell [s]:"; steerDir "Change direction, steerDir"; R "Radius value, R [m]:"; turnDirMask "Turn direction"; cr_ay_max "Lateral acceleration threshold, ay_max [g]:"; cr_ay_stop "Stop simulation at lateral acceleration threshold"; simTime "Simulation time, simTime [s]:"; engine3D "3D Engine"; SceneDesc "Scene:"; dt3D "Engine frame rate, dt3D [s]:"; X_o "Initial longitudinal position, X_o [m]:"; Y_o "Initial lateral position, Y_o [m]:"; Z_o "Initial vertical position, Z_o [m]:"; phi_o "Initial roll angle, phi_o [rad]:"; theta_o "Initial pitch angle, theta_o [rad]:"; psi_o "Initial yaw angle, psi_o [rad]:"
      mask help: Set parameters to configure the maneuver, driver model, and 3D environment. To set the initial vehicle position and orientation, use the parameters on the 3D Engine tab.
      mask init:
      | set_param(gcb,'prevType',get_param(gcb,'manType'))
      settings: AttributesFormatString=%<manType>
      mask Help: eval('vdynblkshelp(''vdcrrefgen'')');
      mask TypeOptions manType: Double Lane Change | Increasing Steer | Swept Sine | Sine with Dwell | Constant Radius
      mask Callback manType:
      | [~]=vdynblksrefconfig(gcb,0);
      | [~]=vdynblksrefconfig(gcb,1);
      mask TypeOptions prevType: Double Lane Change | Increasing Steer | Swept Sine | Sine with Dwell | Constant Radius
      mask TypeOptions xdotUnit: Reference Generator/Double Lane Change/Double Lane Change/xdotUnit | Reference Generator/Constant Radius/xdotUnit | Reference Generator/Increasing Steer/Increasing Steer/xdotUnit | Reference Generator/Sine with Dwell/Sine With Dwell/xdotUnit | Reference Generator/Swept Sine/Swept Sine/xdotUnit
      mask TypeOptions omega_hw: Reference Generator/Increasing Steer/Increasing Steer/omega_hw
      mask TypeOptions theta_max: Reference Generator/Increasing Steer/Increasing Steer/theta_max
      mask TypeOptions t_stop: Reference Generator/Increasing Steer/Increasing Steer/t_stop
      mask TypeOptions ay_max: Reference Generator/Increasing Steer/Increasing Steer/ay_max
      mask TypeOptions ay_stop: Reference Generator/Increasing Steer/Increasing Steer/ay_stop
      mask Callback ay_stop:
      | if strcmp(get_param(gcb,'ay_stop'),'off')
      |     autoblksenableparameters(gcb, [], {'ay_max'},[],[],true);
      | else
      |     autoblksenableparameters(gcb,{'ay_max'},[],[],[],true);
      | end
      mask TypeOptions XGate: Reference Generator/Double Lane Change/Double Lane Change/XGate
      mask TypeOptions xStart: Reference Generator/Double Lane Change/Double Lane Change/xStart
      mask TypeOptions vehW: Reference Generator/Double Lane Change/Double Lane Change/vehW
      mask TypeOptions lattoff: Reference Generator/Double Lane Change/Double Lane Change/lattoff
      mask TypeOptions latRefbp: Reference Generator/Double Lane Change/Double Lane Change/latRefbp
      mask TypeOptions latRef: Reference Generator/Double Lane Change/Double Lane Change/latRef
      mask TypeOptions t_sweep: Reference Generator/Swept Sine/Swept Sine/t_sweep
      mask TypeOptions theta_hw: Reference Generator/Swept Sine/Swept Sine/theta_hw
      mask TypeOptions theta_hw_final: Reference Generator/Swept Sine/Swept Sine/theta_hw_final
      mask TypeOptions steerF: Reference Generator/Sine with Dwell/Sine With Dwell/steerF
      mask TypeOptions steerA: Reference Generator/Sine with Dwell/Sine With Dwell/steerA
      mask TypeOptions tdwell: Reference Generator/Sine with Dwell/Sine With Dwell/tdwell
      mask TypeOptions steerDir: Reference Generator/Sine with Dwell/Sine With Dwell/steerDir
      mask TypeOptions R: Reference Generator/Constant Radius/R
      mask TypeOptions turnDirMask: Reference Generator/Constant Radius/turnDirMask
      mask TypeOptions cr_ay_max: Reference Generator/Constant Radius/ay_max
      mask TypeOptions cr_ay_stop: Reference Generator/Constant Radius/ay_stop
      mask Callback cr_ay_stop:
      | if strcmp(get_param(gcb,'cr_ay_stop'),'off')
      |     autoblksenableparameters(gcb, [], {'cr_ay_max'},[],[],true);
      | else
      |     autoblksenableparameters(gcb,{'cr_ay_max'},[],[],[],true);
      | end
      mask TypeOptions engine3D: 3D Engine/engine3D
      mask TypeOptions SceneDesc: 3D Engine/SceneDesc
      mask Callback SceneDesc: [~] = vdynblks3Dsceneconfig(gcb);
      mask TypeOptions dt3D: 3D Engine/dt3D
      mask TypeOptions defaultPos: Recommended for scene | User-specified
      mask TypeOptions X_o: 3D Engine/X_o
      mask TypeOptions Y_o: 3D Engine/Y_o
      mask TypeOptions Z_o: 3D Engine/Z_o
      mask TypeOptions phi_o: 3D Engine/phi_o
      mask TypeOptions theta_o: 3D Engine/theta_o
      mask TypeOptions psi_o: 3D Engine/psi_o
      mask DialogControl modTab Prompt: Model
      mask DialogControl configGroup Prompt: Configuration
      mask DialogControl ISGroup Prompt: Increasing Steer
      mask DialogControl DLCGroup Prompt: Double Lane Change
      mask DialogControl SSGroup Prompt: Swept Sine
      mask DialogControl SDGroup Prompt: Sine with Dwell
      mask DialogControl CRGroup Prompt: Constant Radius
      mask DialogControl simUpdate Prompt: Set Model Simulation Time
      mask DialogControl simUpdate Callback: [~]=vdynblksrefconfig(gcb,2);
      mask DialogControl sim3DTab Prompt: 3D Engine
      mask DialogControl sim3DGroup Prompt: 3D Engine
      mask DialogControl posSetupDesc Prompt: To use these initial vehicle positions, first Apply the initial values and then click Update the model workspaces with the initial values.
      mask DialogControl setModelPos Prompt: Update model workspaces with initial values
      mask DialogControl setModelPos Callback: [~] = vdynblksmdlWSconfig(gcb);
      mask Display: image('vdbslibscen.png')
  Reshape : Reshape  OutputDimensionality=Customize  OutputDimensions=[2,2]
  SKIDPAD Function : MATLAB Function  TreatAsAtomicUnit=on
  SLALOM Function : MATLAB Function  TreatAsAtomicUnit=on
  Saturation : Saturate  UpperLimit=45  LowerLimit=0
  Saturation1 : Saturate  UpperLimit=45  LowerLimit=0
  Scope{,5,7..8,10..11,13..14,20..21} (10 alike) : Scope
  Scope1 : Scope  NumInputPorts=3
  Scope{2,4,9,12,16,18..19} (7 alike) : Scope  NumInputPorts=2
  Scope15 : Scope  NumInputPorts=4
  Scope17 : Scope  NumInputPorts=4
  Scope3 : Scope  NumInputPorts=3
  Scope6 : Scope  NumInputPorts=3
  Selector : Selector  InputPortWidth=4  IndexOptions=Index vector (dialog)  Indices=[1 2]  OutputSizes=1
  Selector1 : Selector  InputPortWidth=4  IndexOptions=Index vector (dialog)  Indices=[3]  OutputSizes=1
  Selector2 : Selector  InputPortWidth=4  IndexOptions=Index vector (dialog)  Indices=[4]  OutputSizes=1
  Sign : Signum
  Signal Specification : SignalSpecification  Unit=1
  Signal Specification{1..5} (5 alike) : SignalSpecification  Unit=rad/s
  Signal Specification6 : SignalSpecification  Unit=m
  Signal Specification7 : SignalSpecification  Unit=rad
  Signal Specification8 : SignalSpecification  Unit=rad
  Signal Specification9 : SignalSpecification  Unit=rad
  Sum3 : Sum  Inputs=|+-
  Sum4 : Sum  Inputs=-+|
  Sum6 : Sum  Inputs=|+-
  Switch{,1,3..4} (4 alike) : Switch  Criteria=u2 > Threshold
  Switch2 : Switch
  Tempo 1 volta : Display
  Tempo 100m : Display
  Terminator{,1..18,20..21} (21 alike) : Terminator
  Three-axis Inertial Measurement Unit : vehdynlibsens/Three-axis Inertial Measurement Unit  units=Metric (MKS)  imu=[0 0 0]  i_Ts=0  dtype_a=on  w_a=190  z_a=0.707  a_sf_cc=[1 0 0; 0 1 0; 0 0 1]  a_bias=[0 0 0]  a_sat="[-inf  -inf  -inf  inf inf inf]"  dtype_g=on  w_g=19.19  z_g=0.707  g_sf_cc=[1 0 0; 0 1 0; 0 0 1]  g_bias=[0 0 0]  g_sens=[0 0 0]  g_sat="[-inf  -inf  -inf  inf inf inf]"  i_rand=on  i_seeds=[23093 23094 23095 23096 23097 23098]  i_pow=[0.000000007 0.000000007 0.000000007 0.000000007 0.000000007 0.000000007]  aMode=2
      settings: SourceProductBaseCode=VE
  Tire2Veh : Subsystem
  Tires : Subsystem
  Transfer Fcn Filtro APPS : TransferFcn  Numerator=[653594.77124183]  Denominator=[1 1424.8366013072 653594.77124183]
  Transfer Fcn Filtro Volante : TransferFcn  Numerator=[653594.77124183]  Denominator=[1 1424.8366013072 653594.77124183]
  Unit Conversion : UnitConversion
  Unit Conversion1 : UnitConversion
  Vector Concatenate : Concatenate  NumInputs=4
  Vector Concatenate1 : Concatenate  NumInputs=4
  Vector Concatenate10 : Concatenate  NumInputs=3
  Vector Concatenate{2..4,8} (4 alike) : Concatenate
  Vector Concatenate5 : Concatenate  NumInputs=4
  Vector Concatenate6 : Concatenate  NumInputs=3
  Vector Concatenate9 : Concatenate  NumInputs=3
  Veh2Tire : Subsystem
  Vehicle Body 3DOF Dual Track : autolibshared/Vehicle Body 3DOF Single Track  trackMode=Dual  inputMode=External longitudinal forces  frontSteerMode=on  rearSteerMode=off  windMode=on  muMode=on  extFMode=off  extMMode=off  htchFMode=off  htchMMode=off  extXo=off  extpsio=off  extxdoto=off  extro=off  extYo=off  extTamb=off  extydoto=off  aMode=2  NF=EV.NumberOfWheelsPerAxle  NR=EV.NumberOfWheelsPerAxle  m=EV.Mass  a=EV.FrontAxlePositionfromCG  b=EV.RearAxlePositionfromCG  h=EV.HeightCG  dh=1  hh=0.2  X_o=EV.InitialLongPosition  xdot_o=EV.InitialLongVel  CalphaMode=off  sigmaMode=on  d=0  hl=0  w=EV.TrackWidth.*[1 1]  Cy_f=20000  Cy_r=20000  sigma_f=.1  sigma_r=.1  alpha_f_brk=[-.1 .1]  Cy_f_data=[-9e3 9e3]  alpha_r_brk=[-.1 .1]  Cy_r_data=[-9e3 9e3]  Y_o=EV.InitialLatPosition  ydot_o=EV.InitialLatVel  Izz=EV.YawMomentInertia  psi_o=EV.InitialYawAngle  r_o=EV.InitialYawRate  Af=EV.FrontalArea  Cd=EV.LongDragCoeff  Cl=.1  Cpm=.1  beta_w=[0:0.01:0.3]  Cs=[0:0.03:0.9]  Cym=[0:0.01:0.3]  Pabs=101325  Tair=273  g=9.81  mu=1  xdot_tol=1  Fznom=5000  Fxtire_sat=7e3*1e3  Fytire_sat=2e3*1e3  longOff=0  latOff=0  vertOff=.0112  wrapAng=off
      settings: SourceProductBaseCode=PW,DR,MT,UV,VE
  Velocity and Vertical Load : Subsystem  Variant=on  VariantControlMode=label  LabelModeActiveChoice=1
  Visualization : Subsystem
      mask Display: disp('Visualization')
  Wheel Angles : Subsystem
  Wheel Positions : Subsystem
  WheelRadius : Gain  Gain=WHL.LoadedRadius
  le_acelerador : MATLAB Function  TreatAsAtomicUnit=on
  wires:
  Bus Creator5/1 -> [EngTrq], Bus Creator2/1  "Engine"
  Bus Selector8/1 -> Bus Creator/19  "<Beta>"
  Bus Selector1/1 -> Bus to Vector/1
  [Ground] -> For 3D Visualization/3(GroundZ)
  Bus to Vector5/1 -> For 3D Visualization/2(GemoXYZIn)
  Bus Selector9/1 -> Bus to Vector7/1
  Bus Selector7/1 -> Bus to Vector6/1
  Bus to Vector3/1 -> For 3D Visualization/1(angleIn)
  Bus Selector4/1 -> Bus to Vector3/1
  Bus Selector3/1 -> Bus to Vector2/1
  Bus Selector2/1 -> Bus to Vector1/1
  Bus Selector5/1 -> Bus to Vector4/1
  Bus Selector6/1 -> Bus to Vector5/1
  Demux7/3 -> Bus Creator/25  "GeomZdot"
  Demux7/2 -> Bus Creator/24  "GeomYdot"
  Demux7/1 -> Bus Creator/23  "GeomXdot"
  Demux6/3 -> Bus Creator/22  "GeomZ"
  Demux6/2 -> Bus Creator/21  "GeomY"
  Demux6/1 -> Bus Creator/20  "GeomX"
  Demux5/3 -> Bus Creator/18  "az"
  Demux5/2 -> Bus Creator/17  "ay"
  Demux5/1 -> Bus Creator/16  "ax"
  Demux4/3 -> Bus Creator/15  "r"
  Demux4/2 -> Bus Creator/14  "q"
  Demux4/1 -> Bus Creator/13  "p"
  Demux3/3 -> Bus Creator/12  "psi"
  Demux3/2 -> Bus Creator/11  "theta"
  Demux3/1 -> Bus Creator/10  "phi"
  Demux2/3 -> Bus Creator/9  "Zdot"
  Demux2/2 -> Bus Creator/8  "Ydot"
  Demux2/1 -> Bus Creator/7  "Xdot"
  Demux1/3 -> Bus Creator/6  "Z"
  Demux1/2 -> Bus Creator/5  "Y"
  Demux1/1 -> Bus Creator/4  "X"
  Demux/3 -> Bus Creator/3  "zdot"
  Demux/2 -> Bus Creator/2  "ydot"
  Demux/1 -> Scope/1, Bus Creator/1  "xdot"
  For 3D Visualization/2(GeomXYZ) -> Demux6/1
  Bus to Vector6/1 -> Demux7/1
  Bus to Vector2/1 -> Demux5/1
  Bus to Vector4/1 -> Demux4/1
  For 3D Visualization/1(angles) -> Demux3/1
  Bus to Vector1/1 -> Demux2/1
  Bus to Vector/1 -> Demux1/1
  Bus to Vector7/1 -> Demux/1
  Wheel Positions/1(XWheel) -> Bus Creator3/4  "XWheel"
  Wheel Positions/2(YWheel) -> Bus Creator3/5  "YWheel"
  Bus Creator3/1 -> [Wheels]  "Wheels"
  Bus Creator/1 -> Bus Creator2/4  "Chassis"
  Bus Selector13/1 -> Wheel Angles/1(WheelAng), Selector/1  "<WhlAng>"
  Bus Selector13/2 -> Veh2Tire/1(Axle)  "<AxlTrq>"
  [Driveline] -> Bus Selector13/1
  Bus Selector10/4 -> Vector Concatenate1/4  "<G_RR_z>"
  Bus Selector10/3 -> Vector Concatenate1/3  "<G_RL_z>"
  Bus Selector10/2 -> Vector Concatenate1/2  "<G_FR_z>"
  Bus Selector10/1 -> Vector Concatenate1/1  "<G_FL_z>"
  Bus Selector12/4 -> Vector Concatenate/4  "<mu_RR>"
  Bus Selector12/3 -> Vector Concatenate/3  "<mu_RL>"
  Bus Selector12/2 -> Vector Concatenate/2  "<mu_FR>"
  Bus Selector12/1 -> Vector Concatenate/1  "<mu_FL>"
  Bus Selector11/1 -> [Wind]  "<Wind>"
  Environment/1(Env) -> Bus Selector11/1, Bus Selector12/1, Bus Selector10/1
  Axle Forces/2(RearAxlF) -> Vehicle Body 3DOF Dual Track/3
  Axle Forces/1(FrntAxlF) -> Vehicle Body 3DOF Dual Track/2
  Signal Specification/1 -> Vehicle Body 3DOF Dual Track/5
  Vehicle Body 3DOF Dual Track/7 -> Terminator/1
  Vehicle Body 3DOF Dual Track/5 -> Terminator3/1
  Vehicle Body 3DOF Dual Track/4 -> Terminator2/1
  Vehicle Body 3DOF Dual Track/6 -> Terminator1/1
  Vehicle Body 3DOF Dual Track/2 -> Terminator4/1
  Reshape/1 -> Signal Specification/1
  [mu] -> Reshape/1
  Selector/1 -> Vehicle Body 3DOF Dual Track/1
  [EngTrq] -> Bus Selector17/1
  [Wheels] -> Bus Selector15/1
  Bus Selector15/1 -> Selector2/1, Selector1/1  "<omega>"
  Vector Concatenate2/1 -> Vector Concatenate3/1  "FrontWheelAngles"
  Bus Selector14/1 -> Signal Specification9/1  "<Steer>"
  Signal Specification8/1 -> Vector Concatenate2/2  "AngRght"
  Ground3/1 -> Vector Concatenate4/1, Vector Concatenate4/2
  Vector Concatenate4/1 -> Vector Concatenate3/2  "RearWheelAngles"
  Kinematic Steering/1 -> Terminator6/1
  Bus Creator4/1 -> Bus Creator2/3  "Steering"
  Ground/1 -> Bus Creator4/1  "StrWhlTrq"
  Gain/1 -> Signal Specification2/1
  Vector Concatenate3/1 -> Bus Creator1/4  "WhlAng"
  Vector Concatenate5/1 -> Bus Creator1/1  "AxlTrq"
  Bus Creator1/1 -> Bus Creator2/2, [Driveline]  "Driveline"
  Bus Selector18/1 -> Unit Conversion/1  "<LeftMtrSpd>"
  Bus Selector/1 -> Electronic Throttle Actuator Dynamics/1  "<EngTrqCmd>"
  "Mapped Left Motor "/3 -> Gain1/1
  "Mapped Left Motor "/1 -> Terminator8/1
  Unit Conversion/1 -> Signal Specification1/1
  Engine Response/1 -> Bus Creator13/1, Bus Creator5/1  "LeftMtrTrq"
  Selector1/1 -> Gain/1
  Signal Specification2/1 -> Bus Creator1/2  "LeftMtrSpd"
  "Mapped Left Motor "/2 -> Terminator7/1
  Ground2/1 -> Vector Concatenate5/1  "T_FL"
  Bus Selector17/1 -> Vector Concatenate8/1, Vector Concatenate5/3  "<LeftMtrTrq>"
  Ground1/1 -> Vector Concatenate5/2  "T_FR"
  Constant/1 -> "Mapped Left Motor "/1
  [BdyFdbk] -> Bus Selector1/1, Bus Selector3/1, Bus Selector5/1, Bus Selector2/1, Bus Selector9/1
  [BdyFdbk] -> Wheel Positions/1(Info)
  [BdyFdbk] -> Bus Selector8/1, Bus Selector7/1, Bus Selector6/1, Bus Selector4/1
  [Wind] -> Vehicle Body 3DOF Dual Track/4
  [omega] -> Bus Creator3/3
  [kappa] -> Bus Creator3/1
  [alpha] -> Bus Creator3/2
  [dzWheel] -> Bus Creator3/6
  [Wheels] -> Bus Creator2/5
  Tire2Veh/6(alpha) -> [alpha]
  Tire2Veh/5(kappa) -> [kappa]
  Vector Concatenate/1 -> [mu], Scope5/1, Tires/8(lambda)
  Veh2Tire/1(T) -> Tires/1(DriveTorque)
  Velocity and Vertical Load/1(VehV) -> Veh2Tire/3(VehVel)
  Velocity and Vertical Load/2(Fz) -> Tires/7(Fz)
  Veh2Tire/4(psidot) -> Tires/4(r)
  Veh2Tire/5(zdotAxle) -> Terminator9/1
  Bus Selector16/1 -> Veh2Tire/2(r)  "<r>"
  Wheel Angles/1(Vehicle) -> Veh2Tire/4(WheelSteer)
  Constant1/1 -> Tires/6(Press)
  Veh2Tire/2(xdotAxle) -> Tires/2(Vx)  "Vx"
  Tire2Veh/4(omega) -> Signal Specification5/1
  Veh2Tire/3(ydotAxle) -> Tires/3(Vy)  "Vy"
  Tire2Veh/2(FwR) -> Axle Forces/2(R)
  Vector Concatenate1/1 -> [Ground], Tires/9(Gnd)
  Constant3/1 -> Tires/5(Camber), Wheel Angles/2(Camber)
  Vehicle Body 3DOF Dual Track/1 -> [BdyFdbk]
  Tires/1(Out1) -> Tire2Veh/1(Wheel)
  Tire2Veh/1(FwF) -> Axle Forces/1(F)
  Tire2Veh/3(z) -> [dzWheel]
  Constant2/1 -> "Mapped Right Motor "/1
  "Mapped Right Motor "/2 -> Terminator10/1
  "Mapped Right Motor "/1 -> Terminator11/1
  Engine Response1/1 -> Bus Creator13/2, Bus Creator5/2  "RghtMtrTrq"
  Signal Specification1/1 -> "Mapped Left Motor "/2
  "Mapped Right Motor "/3 -> Gain2/1
  Bus Selector17/2 -> Vector Concatenate5/4, Vector Concatenate8/2  "<RghtMtrTrq>"
  Signal Specification3/1 -> Bus Creator1/3  "RghtMtrSpd"
  Selector2/1 -> Gain3/1
  Unit Conversion1/1 -> Signal Specification4/1
  [Driveline] -> Bus Selector18/1
  Bus Selector19/1 -> Unit Conversion1/1  "<RghtMtrSpd>"
  Signal Specification4/1 -> "Mapped Right Motor "/2
  Gain3/1 -> Signal Specification3/1
  Gain1/1 -> Engine Response/1
  Gain2/1 -> Engine Response1/1
  Reference Generator/1(" Vis") -> Visualization/1(Vis)
  Bus Creator10/1 -> Bus Selector/1  "Controller"
  Acc to Torque Request/1 -> Bus Creator9/1, Scope8/1  "EngTrqCmd"
  Bus Creator9/1 -> Bus Creator10/1  "ECU"
  Bus Creator2/1 -> Visualization/3(VehFdbk), [VehFdbk]
  [Driveline] -> Bus Selector19/1
  [Cntrl] -> Visualization/2(Cntrl)
  [VehFdbk] -> Reference Generator/1("VehFdbk ")
  [BdyFdbk] -> Velocity and Vertical Load/1(VehFdbk), Bus Selector16/1
  Signal Specification5/1 -> [omega]
  Vehicle Body 3DOF Dual Track/3 -> Terminator5/1
  Constant14/1 -> Bus Creator11/3  "Brake"
  Constant15/1 -> Bus Creator11/4  "Gear"
  Sum4/1 -> Saturation1/1
  Electronic Throttle Actuator Dynamics/1 -> Sum3/1, Sum4/2
  Sum3/1 -> Saturation/1
  Vector Concatenate8/1 -> Scope7/1
  Saturation1/1 -> "Mapped Right Motor "/3
  Saturation/1 -> "Mapped Left Motor "/3
  Bus Creator13/1 -> Scope13/1  "Engine"
  Entre-Eixos/1 -> Add1/1
  Math Function/1 -> Product/1
  Product/1 -> Add1/2
  Add1/1 -> Divide/2
  Divide/1 -> Product1/2
  Demux9/3 -> Scope20/1, Sum6/2, Scope3/3  "Gyro Yaw"
  Fator de ajustabilidade/1 -> Product2/2
  Sum6/1 -> Scope3/2, [DiferencaYaws]  "Error"
  Demux8/3 -> Terminator17/1
  Demux8/4 -> Terminator16/1
  Demux8/2 -> Scope6/3, Add/2  "FrntRghtWhSpd"
  Add/1 -> Gain9/1
  Gain9/1 -> WheelRadius/1
  Demux8/1 -> Scope6/2, Add/1  "FrntLeftWhlSpd"
  [Wheels] -> Bus Selector32/1
  WheelRadius/1 -> Scope6/1, [FrntAvgSpeed]  "FrntAvgSpeed"
  Bus to Vector8/1 -> Demux8/1
  [FrntAvgSpeed] -> Divide/1, Math Function/1
  Reference Generator/3(" Fdbk") -> Terminator13/1
  Reference Generator/2(" Ref") -> Terminator12/1
  [MaxDesiredYaw] -> Scope3/1, Sum6/1  "Max Desired Yaw"
  Ku/1 -> Product/2
  Switch1/1 -> [RightTorqueVT], Scope2/1  "RightTorqueVT"
  Switch2/1 -> Scope21/1, [LeftTorqueVT], Scope2/2  "LeftTorqueVT"
  Abs/1 -> Switch2/3
  [LeftTorqueVT] -> Sum3/2
  [RightTorqueVT] -> Sum4/1
  Abs1/1 -> Switch1/1
  Signal Specification6/1 -> Distância Percorrida/1, Cálculo do Skidpad/2(Dist)  "Distância Percorrida"
  Integrator1/1 -> Signal Specification6/1
  Bus Selector26/1 -> Cálculo do Slalom/3(Vel), Integrator1/1, Cálculo do Skidpad/3(Vel)  "<xdot>"
  [BdyFdbk] -> Bus Selector26/1
  Cálculo do Skidpad/1(Diam) -> Diâmetro/1
  Kinematic Steering V2/1(AngL) -> Signal Specification7/1  "AngLft"
  Kinematic Steering V2/2(AngR) -> Signal Specification8/1  "AngRght"
  Constant11/1 -> Kinematic Steering V2/2(DadosVolante)
  Constant12/1 -> Kinematic Steering V2/3(DadosE)
  Constant9/1 -> Kinematic Steering V2/4(DadosD)
  Signal Specification7/1 -> Vector Concatenate2/1  "AngLft"
  Signal Specification9/1 -> Kinematic Steering V2/1(Steer)  "Steer"
  AngVolante-> AngRoda/1 -> [AvgWheelSteer], Scope10/1  "AvgWheelSteer"
  le_acelerador/1(acelerador) -> Gain5/1
  [APPS] -> Acc to Torque Request/1
  Gain6/1 -> le_acelerador/1(APPS1)
  "Posição -> Tensão"/1 -> Transfer Fcn Filtro APPS/1
  Transfer Fcn Filtro APPS/1 -> Gain6/1
  [BdyFdbk] -> Bus Selector29/1, Bus Selector27/1, Bus Selector28/1
  Bus Selector27/1 -> Three-axis Inertial Measurement Unit/2  "AngVel"
  Bus Selector28/1 -> Three-axis Inertial Measurement Unit/1  "Acc"
  Bus Selector29/1 -> Three-axis Inertial Measurement Unit/3  "AngAcc"
  Constant13/1 -> Three-axis Inertial Measurement Unit/4
  Constant16/1 -> Three-axis Inertial Measurement Unit/5
  Three-axis Inertial Measurement Unit/1 -> Accelerometer/1, [Accelerometer]
  Three-axis Inertial Measurement Unit/2 -> Gyroscope/1, [Gyroscope]
  [Gyroscope] -> Demux9/1
  Demux9/1 -> Terminator15/1
  Demux9/2 -> Terminator14/1
  Bus Selector25/1 -> Scope4/2, "Posição -> Tensão"/1  "<Accel>"
  Gain5/1 -> Scope4/1, [APPS]
  Transfer Fcn Filtro Volante/1 -> [SteeringWheelSensor]  "SteerSensor"
  Bus Selector23/1 -> Transfer Fcn Filtro Volante/1  "<Steer>"
  [Cntrl] -> Bus Selector25/1, Bus Selector23/1
  [SteeringWheelSensor] -> AngVolante-> AngRoda/1
  Cálculo do Skidpad/2(Temp) -> Tempo 1 volta/1
  Bus Selector32/1 -> Scope14/1, Bus to Vector8/1  "<omega>"
  AccelCmd%/1 -> Bus Creator11/2  "Accel"
  Bus Selector31/1 -> Scope15/1, SLALOM Function/1(X_), Scope17/1, Vector Concatenate9/1  "<X>"
  Bus Selector31/2 -> Scope17/2, Vector Concatenate9/2, Scope15/2, SLALOM Function/2(Y_)  "<Y>"
  Constant22/1 -> Predictive Driver1/3
  [BdyFdbk] -> Bus Selector33/1
  [VehFdbk] -> Bus Selector31/1
  Bus Selector33/1 -> Predictive Driver1/4
  Vector Concatenate9/1 -> Predictive Driver1/5
  SKIDPAD Function/2(y) -> Scope15/4, Vector Concatenate10/2
  Predictive Driver1/3 -> AccelCmd%/1
  Bus Creator11/1 -> [Cntrl], Bus Selector14/1
  Predictive Driver1/2 -> Scope11/1, Bus Creator11/1  "Steer"
  Bus Selector31/3 -> Scope12/1, Scope16/1, Vector Concatenate9/3, SKIDPAD Function/1(psi), SLALOM Function/3(psi)  "<psi>"
  Predictive Driver1/1 -> Terminator20/1
  Predictive Driver1/4 -> Terminator21/1
  SKIDPAD Function/1(x) -> Scope15/3, Vector Concatenate10/1
  Manual Switch/1 -> Predictive Driver1/2
  Vector Concatenate10/1 -> Manual Switch/1
  Vector Concatenate6/1 -> Manual Switch/2
  SLALOM Function/2(y) -> Scope17/4, Vector Concatenate6/2
  SLALOM Function/3(theta) -> Scope16/2, Vector Concatenate6/3
  SKIDPAD Function/3(theta) -> Vector Concatenate10/3, Scope12/2
  SLALOM Function/1(x) -> Scope17/3, Vector Concatenate6/1
  [VehFdbk] -> Bus Selector20/1
  Bus Selector20/1 -> Cálculo do Skidpad/1(Angle)  "<psi>"
  Bus Selector20/2 -> Cálculo do Slalom/2(Y_)  "<Y>"
  Cálculo do Slalom/1(Temp) -> Tempo 100m/1
  Bus Selector20/3 -> Cálculo do Slalom/1(X_)  "<X>"
  Cálculo do Slalom/2(R) -> Raio máximo/1
  [DiferencaYaws] -> Scope19/1, PID Controller1/1
  Manual Switch1/1 -> Abs/1, Switch2/2, Abs1/1, Switch1/2
  Product3/1 -> Divide1/1
  Product2/1 -> Product3/2
  [FrntAvgSpeed] -> Divide1/2
  [AvgWheelSteer] -> Sign/1
  Sign/1 -> Product3/1
  PID Controller1/1 -> Scope19/2, Manual Switch1/1
  [AvgWheelSteer] -> Product1/1
  Ground6/1 -> Manual Switch1/2
  Ground4/1 -> Switch1/3, Switch2/1
  [Driveline] -> Bus Selector21/1
  Bus Selector21/2 -> Product4/2  "<RghtMtrSpd>"
  Constant4/1 -> Product5/2, Product4/1
  Bus Selector21/1 -> Product5/1  "<LeftMtrSpd>"
  Constant5/1 -> Divide2/1
  [FrntAvgSpeed] -> Divide2/2
  Product5/1 -> Product6/1
  Product4/1 -> Product7/1
  Divide2/1 -> Product6/2, Product7/2
  Constant6/1 -> Add3/2, Add4/2
  Product6/1 -> Add3/1
  Product7/1 -> Add4/1
  Constant7/1 -> Product8/1
  Product9/1 -> Math Function1/1
  Constant8/1 -> Product9/1
  [SlipRatio_L] -> Product10/2, Product9/2
  Constant17/1 -> Add5/1
  Math Function1/1 -> Add5/2
  Add5/1 -> Product8/2
  Product8/1 -> Add6/1
  Constant10/1 -> Product10/1
  Product10/1 -> Add6/2
  Add6/1 -> Scope9/1, [Atrito_L]  "Atrito_L"
  Product13/1 -> Math Function2/1
  Constant23/1 -> Product13/1
  Math Function2/1 -> Add7/2
  Constant18/1 -> Product11/1
  Product11/1 -> Add8/2
  Constant19/1 -> Add7/1
  Add7/1 -> Product12/2
  Product12/1 -> Add8/1
  Add8/1 -> Scope9/2, [Atrito_R]  "Atrito_R"
  Constant20/1 -> Product12/1
  [SlipRatio_R] -> Product11/2, Product13/2
  Add4/1 -> Abs5/1
  Abs5/1 -> Scope18/2, [SlipRatio_R]  "SlipRatio_R"
  Add3/1 -> Abs2/1
  Abs2/1 -> Scope18/1, [SlipRatio_L]  "SlipRatio_L"
  [Atrito_L] -> Min1/1
  [Atrito_R] -> Min1/2
  [Atrito] -> Product14/1
  Gravidade/1 -> Product14/2
  Product14/1 -> Product2/1
  Divide1/1 -> Switch3/1, Abs4/1, Scope1/2  "Max Yaw"
  [DesiredYaw] -> Abs3/1, Switch3/3, Scope1/1  "Desired Yaw"
  Abs3/1 -> Add2/1
  Abs4/1 -> Add2/2
  Add2/1 -> Switch3/2
  Switch3/1 -> Scope1/3, [MaxDesiredYaw]
  Product1/1 -> [DesiredYaw]
  Pista seca/1 -> Manual Switch3/1
  Pista molhada/1 -> Manual Switch3/2
  Constant25/1 -> Switch/1
  Constant26/1 -> Switch/3
  Manual Switch3/1 -> Switch4/2, Switch/2
  Switch/1 -> [Atrito]
  Constant24/1 -> Switch4/1
  Constant27/1 -> Switch4/3
  Switch4/1 -> [long_vel]
  [A] -> Predictive Driver1/1
  Min1/1 -> Terminator18/1

== system ContoleLateralApplication_atual/Axle Forces ==
  note: 1) Add Subsystem or Model blocks as valid variant choices.
      | 2) You cannot connect blocks at this level. At simulation, connectivity is automatically
      | determined, based on the active variant and port name matching.
  F : Inport
  R : Inport  Port=2
  Bicycle : Subsystem  VariantControl=0
  Dual : Subsystem  VariantControl=1
  FrntAxlF : Outport  Unit=N  VectorParamsAs1DForOutWhenUnconnected=off
  RearAxlF : Outport  Port=2  Unit=N  VectorParamsAs1DForOutWhenUnconnected=off

== system ContoleLateralApplication_atual/Environment ==
  Bus Creator1 : BusCreator  Inputs=2
  Constant3 : Constant  Value=0
  Constant4 : Constant  Value=0
  Constant5 : Constant  Value=0
  Friction : Constant  Value=GND.Friction
  Ground Feedback : Subsystem  Variant=on  VariantControlMode=label  LabelModeActiveChoice=0
  Vector Concatenate : Concatenate  NumInputs=3
  Env : Outport  VectorParamsAs1DForOutWhenUnconnected=off
  wires:
  Constant5/1 -> Vector Concatenate/3  "Z"
  Vector Concatenate/1 -> Bus Creator1/1  "Wind"
  Constant3/1 -> Vector Concatenate/1  "X"
  Constant4/1 -> Vector Concatenate/2  "Y"
  Ground Feedback/1(Ground) -> Bus Creator1/2  "Gnd"
  Bus Creator1/1 -> Env/1
  Friction/1 -> Ground Feedback/1(Friction)
